simulink model "TLBO_2023"  (R2023b)
settings: Solver=ode45  StartTime=0.0  StopTime=6  MaxStep=1e-4  RelTol=1e-3  EnableMultiTasking=on
PreLoadFcn:
  | Ts_Power=1e-6;
  | Ts_Control=100e-6;
InitFcn:
  | Ts_Power=1e-6;
  | Ts_Control=100e-6;
  | Rtrans=0.142;
  | Xtrans=0.12e-6;
undefined symbols (not defined in the file): DiscIntNeverNeededParam, Ion, Lithium, sigbuilder_block
libraries: dspfdesign x80, spsSeriesRLCBranchLib x52, spsCurrentMeasurementLib x20, spsMeanLib x20, spsIdealSwitchLib x16, spsVoltageMeasurementLib x16, slpidlib x15, spsMosfetLib x14, dspindex x12, spsPWMGeneratorDCDCLib x10, spsGroundLib x10, spsBatteryLib x4
(part 1 of 4)
settings Model: Creator=Philip  LastModifiedBy=LEGION
settings SolverCC: AlgebraicLoopSolver=TrustRegion
settings DataIOCC: ReturnWorkspaceOutputs=off
settings OptimizationCC: LifeSpan=inf
settings DebuggingCC: UnconnectedInputMsg=warning  UnconnectedOutputMsg=warning  UnconnectedLineMsg=warning  SFUnexpectedBacktrackingDiag=warning  SFNoUnconditionalDefaultTransitionDiag=warning  SFExecutionAtInitializationDiag=none  UnderSpecifiedDimensionMsg=warning  ArithmeticOperatorsInVariantConditions=warning
settings ModelReferenceCC: EnableRefExpFcnMdlSchedulingChecks=on
settings SFSimCC: SimUseLocalCustomCode=off  CustomCodeUndefinedFunction=UseInterfaceOnly
settings RTWCC: RTWUseLocalCustomCode=off  DLArmComputeVersion=19.05
settings CodeAppCC: StateflowObjectComments=on
settings GRTTargetCC: TargetLangStandard=C89/C90 (ANSI)
settings ConfigComp: CovMetricSettings=dw  CovSaveCumulativeToWorkspaceVar=on  CovSaveSingleToWorkspaceVar=on  CovExternalEMLEnable=off
settings SimscapeCC: SimscapeNormalizeSystem=off

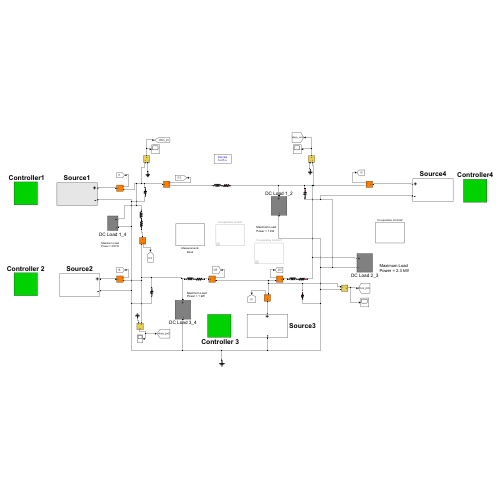
[thumbnail: Simulink's stored preview of the top-level diagram]
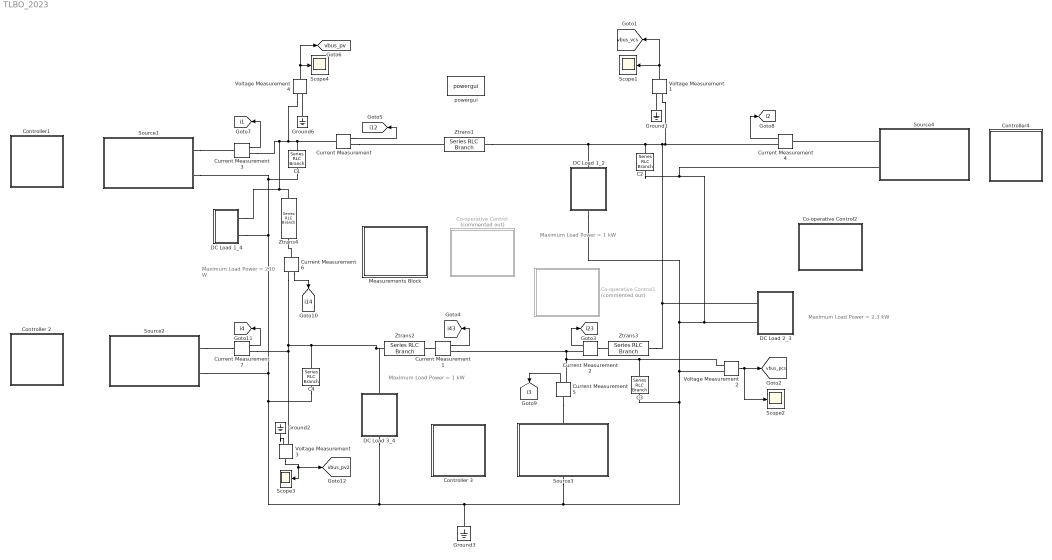
== system TLBO_2023 ==
  note: Maximum Load Power = 1 kW
  note: Maximum Load Power = 230 W
  note: Maximum Load Power = 2.3 kW
  note: Maximum Load Power = 1 kW
  " Controller 3" : Subsystem
  " Controller1" : Subsystem
  C{1..4} (4 alike) : spsSeriesRLCBranchLib/Series RLC Branch  LConnTagsString=__new0  RConnTagsString=__new0  BranchType=C  Resistance=1.0  Inductance=1.0  SetiL0=off  InitialCurrent=0  Capacitance=220e-6  Setx0=off  InitialVoltage=0  Measurements=Branch voltage
  Co-operative Control : Subsystem  Commented=on
  Co-operative Control1 : Subsystem  Commented=on
  Co-operative Control2 : Subsystem
  Controller 2 : Subsystem
  Controller4 : Subsystem
  Current Measurement{,1..7} (8 alike) : spsCurrentMeasurementLib/Current Measurement  PhasorSimulation=off  OutputType=Complex  PSBequivalent=0
  DC Load 1_2 : Subsystem
      settings: PortSchema="{\"entries\":[{\"content\":{\"sides\":[{\"content\":{\"connectorIds\":[]},\"type\":\"ConnectorPlacement.EquallySpacedRectSide\",\"uuid\":\"cddf6359-65bd-4051-86a6-0e07a89083cb\"},{\"content\":{\"connectorIds\":[],\"side\":\"RIGHT\"},\"type\":\"ConnectorPlacement.EquallySpacedRectSide\",\"uuid\":\"60c20b22-281d-4f49-a5be-0230fdaab524\"},{\"content\":{\"connectorIds\":[\"LConn1\"],\"side\":\"TOP\"},\"type\":\"ConnectorPlacement.EquallySpacedRectSide\",\"uuid\":\"1fa402d6-fa22-4172-ba4c-d6acb4a43f4e\"},{\"content\":{\"connectorIds\":[\"RConn1\"],\"side\":\"BOTTOM\"},\"type\":\"ConnectorPlacement.EquallySpacedRectSide\",\"uuid\":\"96e406b9-0d6c-4b79-8101-f8a8e2f9c4fc\"}]},\"type\":\"ConnectorPlacement.EquallySpacedConnector\",\"uuid\":\"d88be4f8-9f42-4009-a911-5cffa4248009\"}],\"packageUris\":[\"http://schema.mathworks.com/mf0/Connector/R2020b\"],\"version\":\"1.0\"}"
  DC Load 1_4 : Subsystem
  DC Load 2_3 : Subsystem
  DC Load 3_4 : Subsystem
      settings: PortSchema="{\"entries\":[{\"content\":{\"sides\":[{\"content\":{\"connectorIds\":[]},\"type\":\"ConnectorPlacement.EquallySpacedRectSide\",\"uuid\":\"cddf6359-65bd-4051-86a6-0e07a89083cb\"},{\"content\":{\"connectorIds\":[],\"side\":\"RIGHT\"},\"type\":\"ConnectorPlacement.EquallySpacedRectSide\",\"uuid\":\"60c20b22-281d-4f49-a5be-0230fdaab524\"},{\"content\":{\"connectorIds\":[\"LConn1\"],\"side\":\"TOP\"},\"type\":\"ConnectorPlacement.EquallySpacedRectSide\",\"uuid\":\"1fa402d6-fa22-4172-ba4c-d6acb4a43f4e\"},{\"content\":{\"connectorIds\":[\"RConn1\"],\"side\":\"BOTTOM\"},\"type\":\"ConnectorPlacement.EquallySpacedRectSide\",\"uuid\":\"96e406b9-0d6c-4b79-8101-f8a8e2f9c4fc\"}]},\"type\":\"ConnectorPlacement.EquallySpacedConnector\",\"uuid\":\"d88be4f8-9f42-4009-a911-5cffa4248009\"}],\"packageUris\":[\"http://schema.mathworks.com/mf0/Connector/R2020b\"],\"version\":\"1.0\"}"
  Ground{1..3,6} (4 alike) : spsGroundLib/Ground  LConnTagsString=a
  Measurements Block : Subsystem
  Scope{1..4} (4 alike) : Scope
  Source1 : Subsystem
  Source2 : Subsystem
  Source3 : Subsystem
  Source4 : Subsystem
  Voltage Measurement{1..4} (4 alike) : spsVoltageMeasurementLib/Voltage Measurement  PhasorSimulation=off  OutputType=Complex  PSBequivalent=0
  Ztrans{1..4} (4 alike) : spsSeriesRLCBranchLib/Series RLC Branch  LConnTagsString=__new0  RConnTagsString=__new0  BranchType=RL  Resistance=Rtrans  Inductance=Xtrans  SetiL0=off  InitialCurrent=0  Capacitance=220e-6  Setx0=off  InitialVoltage=0  Measurements=None
  powergui : spspowerguiLib/powergui  Priority=1  SimulationMode=Discrete  SampleTime=1e-5  frequency=60  Iterations=50  frequencyindice=0  Pbase=100e6  ErrMax=1e-4  UnitsV=kV  UnitsW=MW  buscounter=0  FunctionMessages=off  echomessages=off  EnableUseOfTLC=off  CurrentSourceSwitches=off  DisableSnubberDevices=off  DisableRonSwitches=off  DisableVfSwitches=off  DisplayEquations=off  AutomaticDiscreteSolvers=off  SolverType=Tustin/Backward Euler (TBE)  Interpol=off  ExternalGateDelay=off  methode=off  Ts=100  x0status=blocks  SPID=on  SwTol=0  HookPort=off  NonlinearTolerance=1e-4  nMaxIteration=100  ContinueOnMaxIteration=off  RestoreLinks=warning  ResistiveCurrentMeasurement=off  Frange=[0:2:500]  Ylog=off  Xlog=on  ShowGrid=off  save=off  variable=ZData  structure=0  ZoomFFT=off  StartTime=0.0  cycles=1  DisplayStyle=1  fundamental=60  FreqAxis=off  MaxFrequency=1000  frequencyindicesteady=1  RmsSteady=1  display=off
  tag scope: i12=global, i14=global, i1=global, i23=global, i2=global, i3=global, i43=global, i4=global, vbus_pcs=global, vbus_pv2=global, vbus_pv=global, vbus_vcs=global
  wires:
  Voltage Measurement4/1 -> [vbus_pv], Scope4/1
  Voltage Measurement1/1 -> [vbus_vcs], Scope1/1
  Current Measurement2/1 -> [i23]
  Current Measurement1/1 -> [i43]
  Current Measurement/1 -> [i12]
  Voltage Measurement2/1 -> Scope2/1, [vbus_pcs]
  Current Measurement3/1 -> [i1]
  Current Measurement5/1 -> [i3]
  Current Measurement6/1 -> [i14]
  Current Measurement7/1 -> [i4]
  Voltage Measurement3/1 -> Scope3/1, [vbus_pv2]
  Current Measurement4/1 -> [i2]
  connections:
  Source4/RConn2 -- C2/RConn1 -- Source3/LConn1 -- Ground3/LConn1 -- C4/RConn1 -- C1/RConn1 -- Source1/RConn2 -- DC Load 1_4/LConn2 -- Source2/RConn2 -- DC Load 3_4/RConn1 -- C3/RConn1 -- Voltage Measurement2/LConn2 -- DC Load 1_2/RConn1 -- DC Load 2_3/LConn2
  DC Load 2_3/LConn1 -- Current Measurement4/RConn1 -- Voltage Measurement1/LConn1 -- Ztrans1/LConn1 -- DC Load 1_2/LConn1 -- C2/LConn1 -- Ztrans3/LConn1
  C3/LConn1 -- Voltage Measurement2/LConn1 -- Current Measurement1/RConn1 -- Current Measurement2/RConn1 -- Current Measurement5/RConn1
  Ground6/LConn1 -- Voltage Measurement4/LConn2
  Ground1/LConn1 -- Voltage Measurement1/LConn2
  Current Measurement/RConn1 -- Ztrans1/RConn1
  Current Measurement1/LConn1 -- Ztrans2/LConn1
  Ztrans3/RConn1 -- Current Measurement2/LConn1
  Source1/RConn1 -- Current Measurement3/LConn1
  Source4/RConn1 -- Current Measurement4/LConn1
  Current Measurement5/LConn1 -- Source3/RConn1
  Current Measurement3/RConn1 -- Voltage Measurement4/LConn1 -- Current Measurement/LConn1 -- C1/LConn1 -- Ztrans4/RConn1 -- DC Load 1_4/LConn1
  Current Measurement7/RConn1 -- DC Load 3_4/LConn1 -- Ztrans2/RConn1 -- C4/LConn1 -- Current Measurement6/RConn1 -- Voltage Measurement3/LConn1
  Source2/RConn1 -- Current Measurement7/LConn1
  Ground2/LConn1 -- Voltage Measurement3/LConn2
  Current Measurement6/LConn1 -- Ztrans4/LConn1

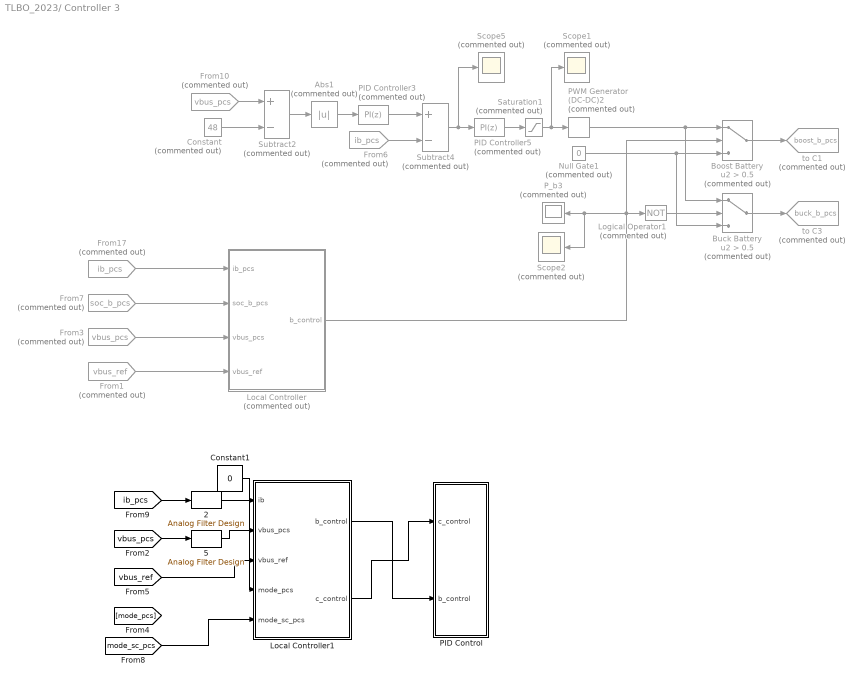
== system TLBO_2023/ Controller 3 ==
  2 : dspfdesign/Analog Filter Design  method=Butterworth  filttype=Lowpass  N=8  Wlo=pi*50  Whi=80  Rp=2  Rs=40
  5 : dspfdesign/Analog Filter Design  method=Butterworth  filttype=Lowpass  N=8  Wlo=pi*50  Whi=80  Rp=2  Rs=40
  Abs1 : Abs  Commented=on  SaturateOnIntegerOverflow=off
  Boost Battery : Switch  Commented=on  Criteria=u2 > Threshold  Threshold=0.5  SaturateOnIntegerOverflow=off  InputSameDT=off
  Buck Battery : Switch  Commented=on  Criteria=u2 > Threshold  Threshold=0.5  SaturateOnIntegerOverflow=off  InputSameDT=off
  Constant : Constant  Commented=on  Value=48
  Constant1 : Constant  Value=0
  From1 : From  Commented=on  GotoTag=vbus_ref  TagVisibility=global
  From10 : From  Commented=on  GotoTag=vbus_pcs  TagVisibility=global
  From17 : From  Commented=on  GotoTag=ib_pcs  TagVisibility=global
  From3 : From  Commented=on  GotoTag=vbus_pcs  TagVisibility=global
  From6 : From  Commented=on  GotoTag=ib_pcs  TagVisibility=global
  From7 : From  Commented=on  GotoTag=soc_b_pcs  TagVisibility=global
  Local Controller : MATLAB Function  Commented=on  TreatAsAtomicUnit=on
  Local Controller1 : MATLAB Function  TreatAsAtomicUnit=on
  Logical Operator1 : Logic  Commented=on  Operator=NOT  AllPortsSameDT=off  OutDataTypeStr=boolean
  Null Gate1 : Constant  Commented=on  Value=0
  PID Control : Subsystem
  PID Controller3 : slpidlib/PID Controller  Commented=on  Controller=PI  Form=Parallel  TimeDomain=Discrete-time  UseExternalTs=off  SampleTime=-1  IntegratorMethod=Forward Euler  FilterMethod=Forward Euler  ControllerParametersSource=internal  P=0  I=4  UseKiTs=off  D=0  N=100  UseFilter=on  TunerSelectOption=Transfer Function Based (PID Tuner App)  InitialConditionSource=internal  InitialConditionForIntegrator=0  InitialConditionForFilter=0  DifferentiatorICPrevScaledInput=0  ExternalReset=none  TrackingMode=off  Kt=1  LimitOutput=off  SatLimitsSource=internal  UpperSaturationLimit=inf  LowerSaturationLimit=-inf  LinearizeAsGain=on  AntiWindupMode=none  Kb=1  LimitIntegrator=off  UpperIntegratorSaturationLimit=inf  LowerIntegratorSaturationLimit=-inf  POutMin=[]  POutMax=[]  IOutMin=[]  IOutMax=[]  DOutMin=[]  DOutMax=[]  NOutMin=[]  NOutMax=[]  SumOutMin=[]  SumOutMax=[]  SaturationOutMin=[]  SaturationOutMax=[]  PParamMin=[]  PParamMax=[]  IParamMin=[]  IParamMax=[]  DParamMin=[]  DParamMax=[]  NParamMin=[]  NParamMax=[]  KbParamMin=[]  KbParamMax=[]  KtParamMin=[]  KtParamMax=[]  KbOutMin=[]  KbOutMax=[]  KtOutMin=[]  KtOutMax=[]  IntegratorOutMin=[]  IntegratorOutMax=[]  FilterOutMin=[]  FilterOutMax=[]  SumI1OutMin=[]  SumI1OutMax=[]  SumI2OutMin=[]  SumI2OutMax=[]  SumI3OutMin=[]  SumI3OutMax=[]  SumI4OutMin=[]  SumI4OutMax=[]  SumDOutMin=[]  SumDOutMax=[]  DifferentiatorOutMin=[]  DifferentiatorOutMax=[]  FilterDiffOutCoefMin=[]  FilterDiffOutCoefMax=[]  ReciprocalOutMin=[]  ReciprocalOutMax=[]  SumDenOutMin=[]  SumDenOutMax=[]  SumNumOutMin=[]  SumNumOutMax=[]  DivideOutMin=[]  DivideOutMax=[]  UdiffTsProdOutMin=[]  UdiffTsProdOutMax=[]  NTsProdOutMin=[]  NTsProdOutMax=[]  UintegralTsProdOutMin=[]  UintegralTsProdOutMax=[]  UngainTsProdOutMin=[]  UngainTsProdOutMax=[]  ClampingZeroOutDataTypeStr=Inherit: Inherit via back propagation  ClampingZeroOutMin=[]  ClampingZeroOutMax=[]  FilterDenConstantOutDataTypeStr=Inherit: Inherit via back propagation  FilterDenConstantOutMin=[]  FilterDenConstantOutMax=[]  PCopyOutDataTypeStr=Inherit: Inherit via back propagation  PCopyOutMin=[]  PCopyOutMax=[]  NCopyOutDataTypeStr=Inherit: Inherit via back propagation  NCopyOutMin=[]  NCopyOutMax=[]  IntegratorContinuousStateAttributes=''  IntegratorStateMustResolveToSignalObject=off  IntegratorRTWStateStorageClass=Auto  FilterContinuousStateAttributes=''  FilterStateMustResolveToSignalObject=off  FilterRTWStateStorageClass=Auto  ParallelPVariant=InternalParameters  IdealPVariant=Disabled  IVariant=InternalParameters  DVariant=Disabled  IntegratorVariant=Discrete  SatVariant=Disabled  AWVariant=Passthrough  PCopyVariant=Disabled  TRVariant=Disabled  FdbkBlocksVariant=Forward  IdealPFdbkVariant=Disabled  SatFdbkVariant=Disabled  DerivativeFilterVariant=Disabled  NVariant=Disabled  NCopyVariant=Disabled_SignalSpec  FilterICVariant=Disabled  IntegratorICVariant=InternalICs  ExternalResetVariant=Disabled  TRSumVariant=Passthrough  SumFdbkVariant=Disabled  SumVariant=Sum_PI  TsampFilterVariant=InternalTs  TsampNgainVariant=Passthrough  TsampIntegralVariant=Disabled_SignalSpec  ExternalSaturationOutDataTypeStr=Inherit: Same as second input
  PID Controller5 : slpidlib/PID Controller  Commented=on  Controller=PI  Form=Parallel  TimeDomain=Discrete-time  UseExternalTs=off  SampleTime=-1  IntegratorMethod=Forward Euler  FilterMethod=Forward Euler  ControllerParametersSource=internal  P=1  I=4  UseKiTs=off  D=1  N=100  UseFilter=on  TunerSelectOption=Transfer Function Based (PID Tuner App)  InitialConditionSource=internal  InitialConditionForIntegrator=0  InitialConditionForFilter=0  DifferentiatorICPrevScaledInput=0  ExternalReset=none  TrackingMode=off  Kt=1  LimitOutput=off  SatLimitsSource=internal  UpperSaturationLimit=inf  LowerSaturationLimit=-inf  LinearizeAsGain=on  AntiWindupMode=none  Kb=1  LimitIntegrator=off  UpperIntegratorSaturationLimit=inf  LowerIntegratorSaturationLimit=-inf  POutMin=[]  POutMax=[]  IOutMin=[]  IOutMax=[]  DOutMin=[]  DOutMax=[]  NOutMin=[]  NOutMax=[]  SumOutMin=[]  SumOutMax=[]  SaturationOutMin=[]  SaturationOutMax=[]  PParamMin=[]  PParamMax=[]  IParamMin=[]  IParamMax=[]  DParamMin=[]  DParamMax=[]  NParamMin=[]  NParamMax=[]  KbParamMin=[]  KbParamMax=[]  KtParamMin=[]  KtParamMax=[]  KbOutMin=[]  KbOutMax=[]  KtOutMin=[]  KtOutMax=[]  IntegratorOutMin=[]  IntegratorOutMax=[]  FilterOutMin=[]  FilterOutMax=[]  SumI1OutMin=[]  SumI1OutMax=[]  SumI2OutMin=[]  SumI2OutMax=[]  SumI3OutMin=[]  SumI3OutMax=[]  SumI4OutMin=[]  SumI4OutMax=[]  SumDOutMin=[]  SumDOutMax=[]  DifferentiatorOutMin=[]  DifferentiatorOutMax=[]  FilterDiffOutCoefMin=[]  FilterDiffOutCoefMax=[]  ReciprocalOutMin=[]  ReciprocalOutMax=[]  SumDenOutMin=[]  SumDenOutMax=[]  SumNumOutMin=[]  SumNumOutMax=[]  DivideOutMin=[]  DivideOutMax=[]  UdiffTsProdOutMin=[]  UdiffTsProdOutMax=[]  NTsProdOutMin=[]  NTsProdOutMax=[]  UintegralTsProdOutMin=[]  UintegralTsProdOutMax=[]  UngainTsProdOutMin=[]  UngainTsProdOutMax=[]  ClampingZeroOutDataTypeStr=Inherit: Inherit via back propagation  ClampingZeroOutMin=[]  ClampingZeroOutMax=[]  FilterDenConstantOutDataTypeStr=Inherit: Inherit via back propagation  FilterDenConstantOutMin=[]  FilterDenConstantOutMax=[]  PCopyOutDataTypeStr=Inherit: Inherit via back propagation  PCopyOutMin=[]  PCopyOutMax=[]  NCopyOutDataTypeStr=Inherit: Inherit via back propagation  NCopyOutMin=[]  NCopyOutMax=[]  IntegratorContinuousStateAttributes=''  IntegratorStateMustResolveToSignalObject=off  IntegratorRTWStateStorageClass=Auto  FilterContinuousStateAttributes=''  FilterStateMustResolveToSignalObject=off  FilterRTWStateStorageClass=Auto  ParallelPVariant=InternalParameters  IdealPVariant=Disabled  IVariant=InternalParameters  DVariant=Disabled  IntegratorVariant=Discrete  SatVariant=Disabled  AWVariant=Passthrough  PCopyVariant=Disabled  TRVariant=Disabled  FdbkBlocksVariant=Forward  IdealPFdbkVariant=Disabled  SatFdbkVariant=Disabled  DerivativeFilterVariant=Disabled  NVariant=Disabled  NCopyVariant=Disabled_SignalSpec  FilterICVariant=Disabled  IntegratorICVariant=InternalICs  ExternalResetVariant=Disabled  TRSumVariant=Passthrough  SumFdbkVariant=Disabled  SumVariant=Sum_PI  TsampFilterVariant=InternalTs  TsampNgainVariant=Passthrough  TsampIntegralVariant=Disabled_SignalSpec  ExternalSaturationOutDataTypeStr=Inherit: Same as second input
  PWM Generator (DC-DC)2 : spsPWMGeneratorDCDCLib/PWM Generator (DC-DC)  Commented=on  Fsw=10e3  Ts=0
  P_b3 : Display  Commented=on
      settings: Format=binary (Stored Integer)  Decimation=1000
  Saturation1 : Saturate  Commented=on  UpperLimit=0.8  LowerLimit=0  ZeroCross=off
  Scope1 : Scope  Commented=on
  Scope2 : Scope  Commented=on
  Scope5 : Scope  Commented=on
  Subtract2 : Sum  Commented=on  Inputs=+-
  Subtract4 : Sum  Commented=on  Inputs=+-
  to C1 : Goto  Commented=on  GotoTag=boost_b_pcs  TagVisibility=global
  to C3 : Goto  Commented=on  GotoTag=buck_b_pcs  TagVisibility=global
  wires:
  Constant/1 -> Subtract2/2
  From1/1 -> Local Controller/4(vbus_ref)
  From6/1 -> Subtract4/2
  PID Controller3/1 -> Subtract4/1
  Subtract4/1 -> PID Controller5/1, Scope5/1
  Saturation1/1 -> PWM Generator (DC-DC)2/1, Scope1/1
  PID Controller5/1 -> Saturation1/1
  PWM Generator (DC-DC)2/1 -> Boost Battery/1, Buck Battery/1
  Abs1/1 -> PID Controller3/1
  From10/1 -> Subtract2/1
  Local Controller/1(b_control) -> Boost Battery/2, Logical Operator1/1, P_b3/1, Scope2/1
  Logical Operator1/1 -> Buck Battery/2
  Subtract2/1 -> Abs1/1
  From7/1 -> Local Controller/2(soc_b_pcs)
  From3/1 -> Local Controller/3(vbus_pcs)
  From17/1 -> Local Controller/1(ib_pcs)
  Null Gate1/1 -> Buck Battery/3, Boost Battery/3
  Boost Battery/1 -> to C1/1
  Buck Battery/1 -> to C3/1
  [vbus_pcs] -> 5/1
  [ib_pcs] -> 2/1
  2/1 -> Local Controller1/1(ib)
  5/1 -> Local Controller1/2(vbus_pcs)
  [vbus_ref] -> Local Controller1/3(vbus_ref)
  Local Controller1/1(b_control) -> PID Control/2(b_control)
  Local Controller1/2(c_control) -> PID Control/1(c_control)
  [mode_sc_pcs] -> Local Controller1/5(mode_sc_pcs)
  Constant1/1 -> Local Controller1/4(mode_pcs)

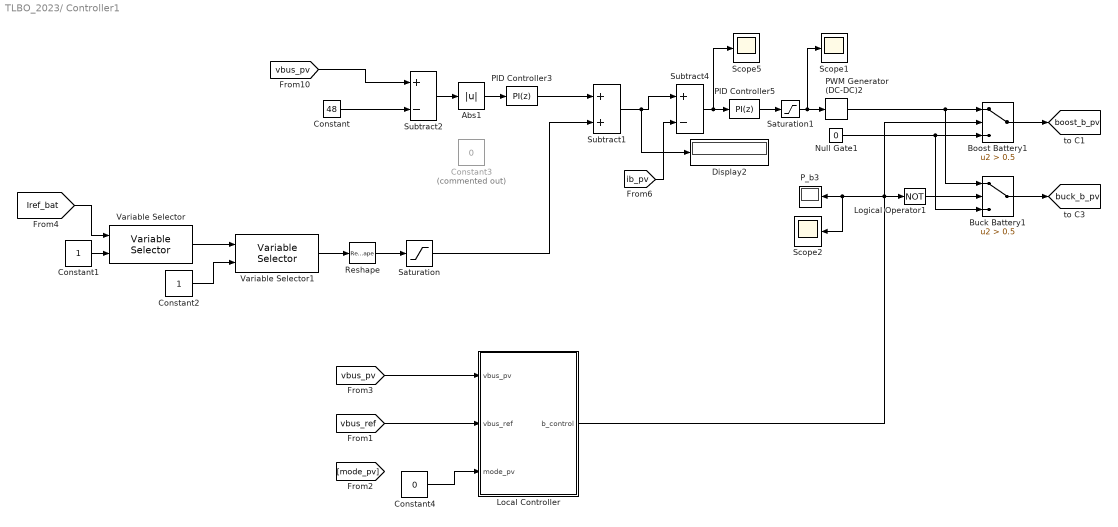
== system TLBO_2023/ Controller1 ==
  Abs1 : Abs  SaturateOnIntegerOverflow=off
  Boost Battery1 : Switch  Criteria=u2 > Threshold  Threshold=0.5  SaturateOnIntegerOverflow=off  InputSameDT=off
  Buck Battery1 : Switch  Criteria=u2 > Threshold  Threshold=0.5  SaturateOnIntegerOverflow=off  InputSameDT=off
  Constant : Constant  Value=48
  Constant1 : Constant
  Constant2 : Constant
  Constant3 : Constant  Commented=on  Value=0
  Constant4 : Constant  Value=0
  Display2 : Display
  Local Controller : MATLAB Function  TreatAsAtomicUnit=on
  Logical Operator1 : Logic  Operator=NOT  AllPortsSameDT=off  OutDataTypeStr=boolean
  Null Gate1 : Constant  Value=0
  PID Controller3 : slpidlib/PID Controller  Controller=PI  Form=Parallel  TimeDomain=Discrete-time  UseExternalTs=off  SampleTime=-1  IntegratorMethod=Forward Euler  FilterMethod=Forward Euler  ControllerParametersSource=internal  P=0  I=4  UseKiTs=off  D=0  N=100  UseFilter=on  TunerSelectOption=Transfer Function Based (PID Tuner App)  InitialConditionSource=internal  InitialConditionForIntegrator=0  InitialConditionForFilter=0  DifferentiatorICPrevScaledInput=0  ExternalReset=none  TrackingMode=off  Kt=1  LimitOutput=off  SatLimitsSource=internal  UpperSaturationLimit=inf  LowerSaturationLimit=-inf  LinearizeAsGain=on  AntiWindupMode=none  Kb=1  LimitIntegrator=off  UpperIntegratorSaturationLimit=inf  LowerIntegratorSaturationLimit=-inf  POutMin=[]  POutMax=[]  IOutMin=[]  IOutMax=[]  DOutMin=[]  DOutMax=[]  NOutMin=[]  NOutMax=[]  SumOutMin=[]  SumOutMax=[]  SaturationOutMin=[]  SaturationOutMax=[]  PParamMin=[]  PParamMax=[]  IParamMin=[]  IParamMax=[]  DParamMin=[]  DParamMax=[]  NParamMin=[]  NParamMax=[]  KbParamMin=[]  KbParamMax=[]  KtParamMin=[]  KtParamMax=[]  KbOutMin=[]  KbOutMax=[]  KtOutMin=[]  KtOutMax=[]  IntegratorOutMin=[]  IntegratorOutMax=[]  FilterOutMin=[]  FilterOutMax=[]  SumI1OutMin=[]  SumI1OutMax=[]  SumI2OutMin=[]  SumI2OutMax=[]  SumI3OutMin=[]  SumI3OutMax=[]  SumI4OutMin=[]  SumI4OutMax=[]  SumDOutMin=[]  SumDOutMax=[]  DifferentiatorOutMin=[]  DifferentiatorOutMax=[]  FilterDiffOutCoefMin=[]  FilterDiffOutCoefMax=[]  ReciprocalOutMin=[]  ReciprocalOutMax=[]  SumDenOutMin=[]  SumDenOutMax=[]  SumNumOutMin=[]  SumNumOutMax=[]  DivideOutMin=[]  DivideOutMax=[]  UdiffTsProdOutMin=[]  UdiffTsProdOutMax=[]  NTsProdOutMin=[]  NTsProdOutMax=[]  UintegralTsProdOutMin=[]  UintegralTsProdOutMax=[]  UngainTsProdOutMin=[]  UngainTsProdOutMax=[]  ClampingZeroOutDataTypeStr=Inherit: Inherit via back propagation  ClampingZeroOutMin=[]  ClampingZeroOutMax=[]  FilterDenConstantOutDataTypeStr=Inherit: Inherit via back propagation  FilterDenConstantOutMin=[]  FilterDenConstantOutMax=[]  PCopyOutDataTypeStr=Inherit: Inherit via back propagation  PCopyOutMin=[]  PCopyOutMax=[]  NCopyOutDataTypeStr=Inherit: Inherit via back propagation  NCopyOutMin=[]  NCopyOutMax=[]  IntegratorContinuousStateAttributes=''  IntegratorStateMustResolveToSignalObject=off  IntegratorRTWStateStorageClass=Auto  FilterContinuousStateAttributes=''  FilterStateMustResolveToSignalObject=off  FilterRTWStateStorageClass=Auto  ParallelPVariant=InternalParameters  IdealPVariant=Disabled  IVariant=InternalParameters  DVariant=Disabled  IntegratorVariant=Discrete  SatVariant=Disabled  AWVariant=Passthrough  PCopyVariant=Disabled  TRVariant=Disabled  FdbkBlocksVariant=Forward  IdealPFdbkVariant=Disabled  SatFdbkVariant=Disabled  DerivativeFilterVariant=Disabled  NVariant=Disabled  NCopyVariant=Disabled_SignalSpec  FilterICVariant=Disabled  IntegratorICVariant=InternalICs  ExternalResetVariant=Disabled  TRSumVariant=Passthrough  SumFdbkVariant=Disabled  SumVariant=Sum_PI  TsampFilterVariant=InternalTs  TsampNgainVariant=Passthrough  TsampIntegralVariant=Disabled_SignalSpec  ExternalSaturationOutDataTypeStr=Inherit: Same as second input
  PID Controller5 : slpidlib/PID Controller  Controller=PI  Form=Parallel  TimeDomain=Discrete-time  UseExternalTs=off  SampleTime=-1  IntegratorMethod=Forward Euler  FilterMethod=Forward Euler  ControllerParametersSource=internal  P=10  I=4  UseKiTs=off  D=10  N=100  UseFilter=on  TunerSelectOption=Transfer Function Based (PID Tuner App)  InitialConditionSource=internal  InitialConditionForIntegrator=0  InitialConditionForFilter=0  DifferentiatorICPrevScaledInput=0  ExternalReset=none  TrackingMode=off  Kt=1  LimitOutput=off  SatLimitsSource=internal  UpperSaturationLimit=inf  LowerSaturationLimit=-inf  LinearizeAsGain=on  AntiWindupMode=none  Kb=1  LimitIntegrator=off  UpperIntegratorSaturationLimit=inf  LowerIntegratorSaturationLimit=-inf  POutMin=[]  POutMax=[]  IOutMin=[]  IOutMax=[]  DOutMin=[]  DOutMax=[]  NOutMin=[]  NOutMax=[]  SumOutMin=[]  SumOutMax=[]  SaturationOutMin=[]  SaturationOutMax=[]  PParamMin=[]  PParamMax=[]  IParamMin=[]  IParamMax=[]  DParamMin=[]  DParamMax=[]  NParamMin=[]  NParamMax=[]  KbParamMin=[]  KbParamMax=[]  KtParamMin=[]  KtParamMax=[]  KbOutMin=[]  KbOutMax=[]  KtOutMin=[]  KtOutMax=[]  IntegratorOutMin=[]  IntegratorOutMax=[]  FilterOutMin=[]  FilterOutMax=[]  SumI1OutMin=[]  SumI1OutMax=[]  SumI2OutMin=[]  SumI2OutMax=[]  SumI3OutMin=[]  SumI3OutMax=[]  SumI4OutMin=[]  SumI4OutMax=[]  SumDOutMin=[]  SumDOutMax=[]  DifferentiatorOutMin=[]  DifferentiatorOutMax=[]  FilterDiffOutCoefMin=[]  FilterDiffOutCoefMax=[]  ReciprocalOutMin=[]  ReciprocalOutMax=[]  SumDenOutMin=[]  SumDenOutMax=[]  SumNumOutMin=[]  SumNumOutMax=[]  DivideOutMin=[]  DivideOutMax=[]  UdiffTsProdOutMin=[]  UdiffTsProdOutMax=[]  NTsProdOutMin=[]  NTsProdOutMax=[]  UintegralTsProdOutMin=[]  UintegralTsProdOutMax=[]  UngainTsProdOutMin=[]  UngainTsProdOutMax=[]  ClampingZeroOutDataTypeStr=Inherit: Inherit via back propagation  ClampingZeroOutMin=[]  ClampingZeroOutMax=[]  FilterDenConstantOutDataTypeStr=Inherit: Inherit via back propagation  FilterDenConstantOutMin=[]  FilterDenConstantOutMax=[]  PCopyOutDataTypeStr=Inherit: Inherit via back propagation  PCopyOutMin=[]  PCopyOutMax=[]  NCopyOutDataTypeStr=Inherit: Inherit via back propagation  NCopyOutMin=[]  NCopyOutMax=[]  IntegratorContinuousStateAttributes=''  IntegratorStateMustResolveToSignalObject=off  IntegratorRTWStateStorageClass=Auto  FilterContinuousStateAttributes=''  FilterStateMustResolveToSignalObject=off  FilterRTWStateStorageClass=Auto  ParallelPVariant=InternalParameters  IdealPVariant=Disabled  IVariant=InternalParameters  DVariant=Disabled  IntegratorVariant=Discrete  SatVariant=Disabled  AWVariant=Passthrough  PCopyVariant=Disabled  TRVariant=Disabled  FdbkBlocksVariant=Forward  IdealPFdbkVariant=Disabled  SatFdbkVariant=Disabled  DerivativeFilterVariant=Disabled  NVariant=Disabled  NCopyVariant=Disabled_SignalSpec  FilterICVariant=Disabled  IntegratorICVariant=InternalICs  ExternalResetVariant=Disabled  TRSumVariant=Passthrough  SumFdbkVariant=Disabled  SumVariant=Sum_PI  TsampFilterVariant=InternalTs  TsampNgainVariant=Passthrough  TsampIntegralVariant=Disabled_SignalSpec  ExternalSaturationOutDataTypeStr=Inherit: Same as second input
  PWM Generator (DC-DC)2 : spsPWMGeneratorDCDCLib/PWM Generator (DC-DC)  Fsw=10e3  Ts=0
  P_b3 : Display
      settings: Format=binary (Stored Integer)  Decimation=1000
  Reshape : Reshape
  Saturation : Saturate
  Saturation1 : Saturate  UpperLimit=0.8  LowerLimit=0  ZeroCross=off
  Scope1 : Scope
  Scope2 : Scope
  Scope5 : Scope
  Subtract1 : Sum
  Subtract2 : Sum  Inputs=+-
  Subtract4 : Sum  Inputs=+-
  Variable Selector : dspindex/Variable Selector  NumInputs=1  rowsOrCols=Rows  IdxMode=Variable  Elements=[1 3]  ZerOneIdxMode=One-based  errmode=Clip Index  FillMode=on  FillValues=0
  Variable Selector1 : dspindex/Variable Selector  NumInputs=1  rowsOrCols=Columns  IdxMode=Variable  Elements=[1 3]  ZerOneIdxMode=One-based  errmode=Clip Index  FillMode=on  FillValues=0
  tag scope: boost_b_pv=global, buck_b_pv=global
  wires:
  Buck Battery1/1 -> [buck_b_pv]
  Boost Battery1/1 -> [boost_b_pv]
  Null Gate1/1 -> Boost Battery1/3, Buck Battery1/3
  [vbus_pv] -> Local Controller/1(vbus_pv)
  Subtract2/1 -> Abs1/1
  Logical Operator1/1 -> Buck Battery1/2
  Local Controller/1(b_control) -> Scope2/1, P_b3/1, Logical Operator1/1, Boost Battery1/2
  Abs1/1 -> PID Controller3/1
  PWM Generator (DC-DC)2/1 -> Buck Battery1/1, Boost Battery1/1
  PID Controller5/1 -> Saturation1/1
  Saturation1/1 -> Scope1/1, PWM Generator (DC-DC)2/1
  Subtract4/1 -> Scope5/1, PID Controller5/1
  [vbus_ref] -> Local Controller/2(vbus_ref)
  [ib_pv] -> Subtract4/2
  [vbus_pv] -> Subtract2/1
  [Iref_bat] -> Variable Selector/1
  Constant1/1 -> Variable Selector/2
  Variable Selector/1 -> Variable Selector1/1
  Constant2/1 -> Variable Selector1/2
  Constant/1 -> Subtract2/2
  Variable Selector1/1 -> Reshape/1
  PID Controller3/1 -> Subtract1/1
  Subtract1/1 -> Display2/1, Subtract4/1
  Reshape/1 -> Saturation/1
  Saturation/1 -> Subtract1/2
  Constant4/1 -> Local Controller/3(mode_pv)

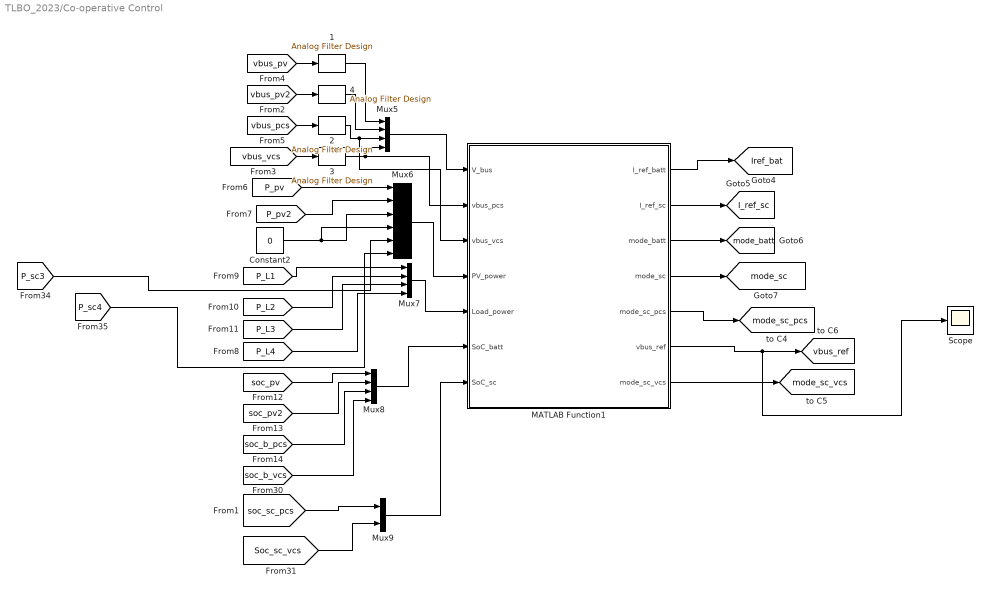
== system TLBO_2023/Co-operative Control ==
  {1..4} (4 alike) : dspfdesign/Analog Filter Design  method=Butterworth  filttype=Lowpass  N=8  Wlo=pi*50  Whi=80  Rp=2  Rs=40
  Constant2 : Constant  Value=0
  MATLAB Function1 : MATLAB Function  TreatAsAtomicUnit=on
  Mux5 : Mux
  Mux6 : Mux  Inputs=6
  Mux7 : Mux
  Mux8 : Mux
  Mux9 : Mux  Inputs=2
  Scope : Scope
  tag scope: I_ref_sc=global, Iref_bat=global, mode_batt=global, mode_sc=global, mode_sc_pcs=global, mode_sc_vcs=global, vbus_ref=global
  wires:
  Mux5/1 -> MATLAB Function1/1(V_bus)
  [P_L1] -> Mux7/1
  [Soc_sc_vcs] -> Mux9/2
  Constant2/1 -> Mux6/3, Mux6/4
  [P_pv2] -> Mux6/2
  Mux8/1 -> MATLAB Function1/6(SoC_batt)
  [soc_b_vcs] -> Mux8/4
  [vbus_pv2] -> 4/1
  [P_pv] -> Mux6/1
  [soc_pv2] -> Mux8/2
  [vbus_vcs] -> 3/1
  2/1 -> MATLAB Function1/3(vbus_vcs), Mux5/3
  [vbus_pcs] -> 2/1
  [soc_sc_pcs] -> Mux9/1
  [P_L3] -> Mux7/3
  3/1 -> MATLAB Function1/2(vbus_pcs), Mux5/4
  [vbus_pv] -> 1/1
  Mux9/1 -> MATLAB Function1/7(SoC_sc)
  [P_L2] -> Mux7/2
  [soc_b_pcs] -> Mux8/3
  1/1 -> Mux5/1
  [soc_pv] -> Mux8/1
  Mux6/1 -> MATLAB Function1/4(PV_power)
  Mux7/1 -> MATLAB Function1/5(Load_power)
  [P_L4] -> Mux7/4
  4/1 -> Mux5/2
  MATLAB Function1/1(I_ref_batt) -> [Iref_bat]
  [P_sc4] -> Mux6/6
  [P_sc3] -> Mux6/5
  MATLAB Function1/2(I_ref_sc) -> [I_ref_sc]
  MATLAB Function1/3(mode_batt) -> [mode_batt]
  MATLAB Function1/4(mode_sc) -> [mode_sc]
  MATLAB Function1/5(mode_sc_pcs) -> [mode_sc_pcs]
  MATLAB Function1/7(mode_sc_vcs) -> [mode_sc_vcs]
  MATLAB Function1/6(vbus_ref) -> Scope/1, [vbus_ref]

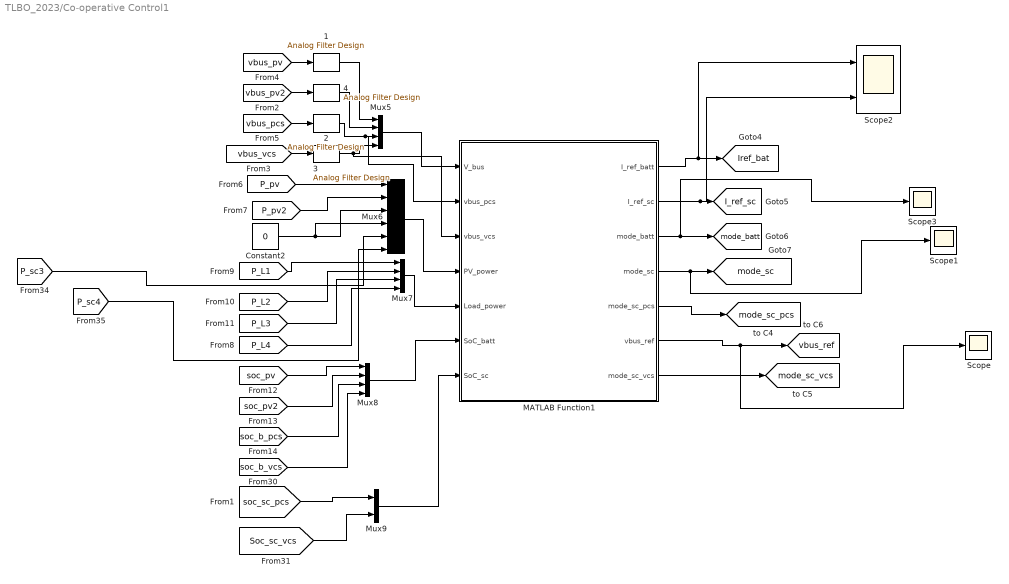
== system TLBO_2023/Co-operative Control1 ==
  {1..4} (4 alike) : dspfdesign/Analog Filter Design  method=Butterworth  filttype=Lowpass  N=8  Wlo=pi*50  Whi=80  Rp=2  Rs=40
  Constant2 : Constant  Value=0
  MATLAB Function1 : MATLAB Function  TreatAsAtomicUnit=on
  Mux5 : Mux
  Mux6 : Mux  Inputs=6
  Mux7 : Mux
  Mux8 : Mux
  Mux9 : Mux  Inputs=2
  Scope : Scope
  Scope1 : Scope
  Scope2 : Scope  NumInputPorts=2
  Scope3 : Scope
  tag scope: I_ref_sc=global, Iref_bat=global, mode_batt=global, mode_sc=global, mode_sc_pcs=global, mode_sc_vcs=global, vbus_ref=global
  wires:
  MATLAB Function1/6(vbus_ref) -> Scope/1, [vbus_ref]
  MATLAB Function1/7(mode_sc_vcs) -> [mode_sc_vcs]
  MATLAB Function1/5(mode_sc_pcs) -> [mode_sc_pcs]
  MATLAB Function1/4(mode_sc) -> Scope1/1, [mode_sc]
  MATLAB Function1/3(mode_batt) -> Scope3/1, [mode_batt]
  MATLAB Function1/2(I_ref_sc) -> Scope2/2, [I_ref_sc]
  [P_sc3] -> Mux6/5
  [P_sc4] -> Mux6/6
  MATLAB Function1/1(I_ref_batt) -> Scope2/1, [Iref_bat]
  4/1 -> Mux5/2
  [P_L4] -> Mux7/4
  [soc_pv] -> Mux8/1
  1/1 -> Mux5/1
  [soc_b_pcs] -> Mux8/3
  [P_L2] -> Mux7/2
  [vbus_pv] -> 1/1
  3/1 -> MATLAB Function1/3(vbus_vcs), Mux5/4
  [P_L3] -> Mux7/3
  [soc_sc_pcs] -> Mux9/1
  [vbus_pcs] -> 2/1
  2/1 -> MATLAB Function1/2(vbus_pcs), Mux5/3
  [vbus_vcs] -> 3/1
  [soc_pv2] -> Mux8/2
  [P_pv] -> Mux6/1
  [vbus_pv2] -> 4/1
  [soc_b_vcs] -> Mux8/4
  [P_pv2] -> Mux6/2
  Constant2/1 -> Mux6/4, Mux6/3
  [Soc_sc_vcs] -> Mux9/2
  [P_L1] -> Mux7/1
  Mux5/1 -> MATLAB Function1/1(V_bus)
  Mux6/1 -> MATLAB Function1/4(PV_power)
  Mux7/1 -> MATLAB Function1/5(Load_power)
  Mux8/1 -> MATLAB Function1/6(SoC_batt)
  Mux9/1 -> MATLAB Function1/7(SoC_sc)

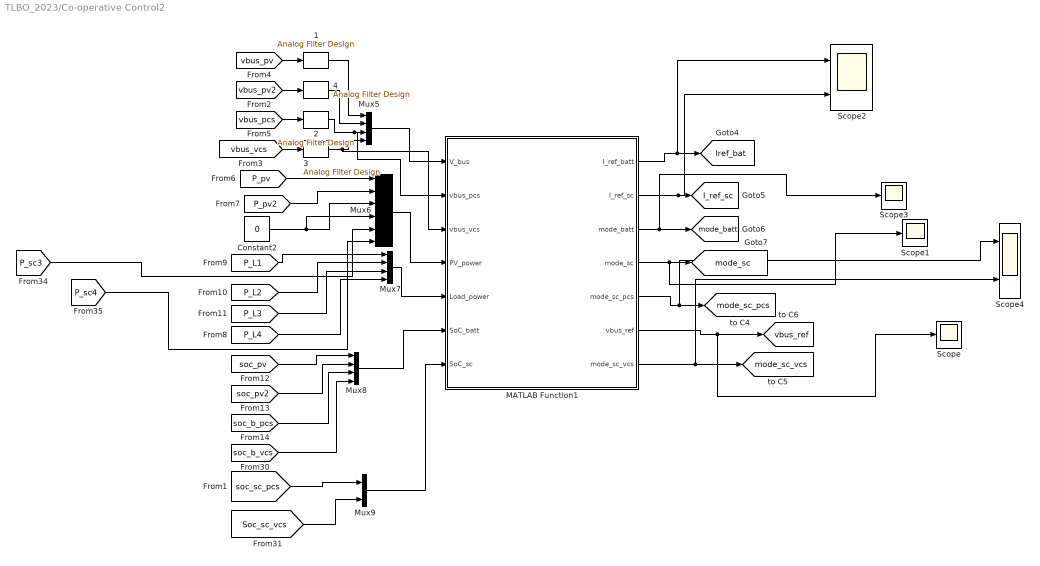
== system TLBO_2023/Co-operative Control2 ==
  {1..4} (4 alike) : dspfdesign/Analog Filter Design  method=Butterworth  filttype=Lowpass  N=8  Wlo=pi*50  Whi=80  Rp=2  Rs=40
  Constant2 : Constant  Value=0
  MATLAB Function1 : MATLAB Function  TreatAsAtomicUnit=on
  Mux5 : Mux
  Mux6 : Mux  Inputs=6
  Mux7 : Mux
  Mux8 : Mux
  Mux9 : Mux  Inputs=2
  Scope : Scope
  Scope1 : Scope
  Scope2 : Scope  NumInputPorts=2
  Scope3 : Scope
  Scope4 : Scope  NumInputPorts=2
  tag scope: I_ref_sc=global, Iref_bat=global, mode_batt=global, mode_sc=global, mode_sc_pcs=global, mode_sc_vcs=global, vbus_ref=global
  wires:
  Mux9/1 -> MATLAB Function1/7(SoC_sc)
  Mux8/1 -> MATLAB Function1/6(SoC_batt)
  Mux7/1 -> MATLAB Function1/5(Load_power)
  Mux6/1 -> MATLAB Function1/4(PV_power)
  Mux5/1 -> MATLAB Function1/1(V_bus)
  [P_L1] -> Mux7/1
  [Soc_sc_vcs] -> Mux9/2
  Constant2/1 -> Mux6/3, Mux6/4
  [P_pv2] -> Mux6/2
  [soc_b_vcs] -> Mux8/4
  [vbus_pv2] -> 4/1
  [P_pv] -> Mux6/1
  [soc_pv2] -> Mux8/2
  [vbus_vcs] -> 3/1
  2/1 -> Mux5/3, MATLAB Function1/2(vbus_pcs)
  [vbus_pcs] -> 2/1
  [soc_sc_pcs] -> Mux9/1
  [P_L3] -> Mux7/3
  3/1 -> Mux5/4, MATLAB Function1/3(vbus_vcs)
  [vbus_pv] -> 1/1
  [P_L2] -> Mux7/2
  [soc_b_pcs] -> Mux8/3
  1/1 -> Mux5/1
  [soc_pv] -> Mux8/1
  [P_L4] -> Mux7/4
  4/1 -> Mux5/2
  MATLAB Function1/1(I_ref_batt) -> [Iref_bat], Scope2/1
  [P_sc4] -> Mux6/6
  [P_sc3] -> Mux6/5
  MATLAB Function1/2(I_ref_sc) -> [I_ref_sc], Scope2/2
  MATLAB Function1/3(mode_batt) -> [mode_batt], Scope3/1
  MATLAB Function1/4(mode_sc) -> [mode_sc], Scope1/1
  MATLAB Function1/5(mode_sc_pcs) -> Scope4/1, [mode_sc_pcs]
  MATLAB Function1/7(mode_sc_vcs) -> Scope4/2, [mode_sc_vcs]
  MATLAB Function1/6(vbus_ref) -> [vbus_ref], Scope/1

== system TLBO_2023/Controller 2 ==
  Abs1 : Abs  SaturateOnIntegerOverflow=off
  Boost Battery1 : Switch  Criteria=u2 > Threshold  Threshold=0.5  SaturateOnIntegerOverflow=off  InputSameDT=off
  Buck Battery1 : Switch  Criteria=u2 > Threshold  Threshold=0.5  SaturateOnIntegerOverflow=off  InputSameDT=off
  Constant : Constant  Value=48
  Constant1 : Constant
  Constant2 : Constant  Value=2
  Constant3 : Constant  Value=0
  Constant4 : Constant  Value=0
  Local Controller : MATLAB Function  TreatAsAtomicUnit=on
  Logical Operator1 : Logic  Operator=NOT  AllPortsSameDT=off  OutDataTypeStr=boolean
  Null Gate1 : Constant  Value=0
  PID Controller3 : slpidlib/PID Controller  Controller=PI  Form=Parallel  TimeDomain=Discrete-time  UseExternalTs=off  SampleTime=-1  IntegratorMethod=Forward Euler  FilterMethod=Forward Euler  ControllerParametersSource=internal  P=0  I=4  UseKiTs=off  D=0  N=100  UseFilter=on  TunerSelectOption=Transfer Function Based (PID Tuner App)  InitialConditionSource=internal  InitialConditionForIntegrator=0  InitialConditionForFilter=0  DifferentiatorICPrevScaledInput=0  ExternalReset=none  TrackingMode=off  Kt=1  LimitOutput=off  SatLimitsSource=internal  UpperSaturationLimit=inf  LowerSaturationLimit=-inf  LinearizeAsGain=on  AntiWindupMode=none  Kb=1  LimitIntegrator=off  UpperIntegratorSaturationLimit=inf  LowerIntegratorSaturationLimit=-inf  POutMin=[]  POutMax=[]  IOutMin=[]  IOutMax=[]  DOutMin=[]  DOutMax=[]  NOutMin=[]  NOutMax=[]  SumOutMin=[]  SumOutMax=[]  SaturationOutMin=[]  SaturationOutMax=[]  PParamMin=[]  PParamMax=[]  IParamMin=[]  IParamMax=[]  DParamMin=[]  DParamMax=[]  NParamMin=[]  NParamMax=[]  KbParamMin=[]  KbParamMax=[]  KtParamMin=[]  KtParamMax=[]  KbOutMin=[]  KbOutMax=[]  KtOutMin=[]  KtOutMax=[]  IntegratorOutMin=[]  IntegratorOutMax=[]  FilterOutMin=[]  FilterOutMax=[]  SumI1OutMin=[]  SumI1OutMax=[]  SumI2OutMin=[]  SumI2OutMax=[]  SumI3OutMin=[]  SumI3OutMax=[]  SumI4OutMin=[]  SumI4OutMax=[]  SumDOutMin=[]  SumDOutMax=[]  DifferentiatorOutMin=[]  DifferentiatorOutMax=[]  FilterDiffOutCoefMin=[]  FilterDiffOutCoefMax=[]  ReciprocalOutMin=[]  ReciprocalOutMax=[]  SumDenOutMin=[]  SumDenOutMax=[]  SumNumOutMin=[]  SumNumOutMax=[]  DivideOutMin=[]  DivideOutMax=[]  UdiffTsProdOutMin=[]  UdiffTsProdOutMax=[]  NTsProdOutMin=[]  NTsProdOutMax=[]  UintegralTsProdOutMin=[]  UintegralTsProdOutMax=[]  UngainTsProdOutMin=[]  UngainTsProdOutMax=[]  ClampingZeroOutDataTypeStr=Inherit: Inherit via back propagation  ClampingZeroOutMin=[]  ClampingZeroOutMax=[]  FilterDenConstantOutDataTypeStr=Inherit: Inherit via back propagation  FilterDenConstantOutMin=[]  FilterDenConstantOutMax=[]  PCopyOutDataTypeStr=Inherit: Inherit via back propagation  PCopyOutMin=[]  PCopyOutMax=[]  NCopyOutDataTypeStr=Inherit: Inherit via back propagation  NCopyOutMin=[]  NCopyOutMax=[]  IntegratorContinuousStateAttributes=''  IntegratorStateMustResolveToSignalObject=off  IntegratorRTWStateStorageClass=Auto  FilterContinuousStateAttributes=''  FilterStateMustResolveToSignalObject=off  FilterRTWStateStorageClass=Auto  ParallelPVariant=InternalParameters  IdealPVariant=Disabled  IVariant=InternalParameters  DVariant=Disabled  IntegratorVariant=Discrete  SatVariant=Disabled  AWVariant=Passthrough  PCopyVariant=Disabled  TRVariant=Disabled  FdbkBlocksVariant=Forward  IdealPFdbkVariant=Disabled  SatFdbkVariant=Disabled  DerivativeFilterVariant=Disabled  NVariant=Disabled  NCopyVariant=Disabled_SignalSpec  FilterICVariant=Disabled  IntegratorICVariant=InternalICs  ExternalResetVariant=Disabled  TRSumVariant=Passthrough  SumFdbkVariant=Disabled  SumVariant=Sum_PI  TsampFilterVariant=InternalTs  TsampNgainVariant=Passthrough  TsampIntegralVariant=Disabled_SignalSpec  ExternalSaturationOutDataTypeStr=Inherit: Same as second input
  PID Controller5 : slpidlib/PID Controller  Controller=PI  Form=Parallel  TimeDomain=Discrete-time  UseExternalTs=off  SampleTime=-1  IntegratorMethod=Forward Euler  FilterMethod=Forward Euler  ControllerParametersSource=internal  P=10  I=4  UseKiTs=off  D=10  N=100  UseFilter=on  TunerSelectOption=Transfer Function Based (PID Tuner App)  InitialConditionSource=internal  InitialConditionForIntegrator=0  InitialConditionForFilter=0  DifferentiatorICPrevScaledInput=0  ExternalReset=none  TrackingMode=off  Kt=1  LimitOutput=off  SatLimitsSource=internal  UpperSaturationLimit=inf  LowerSaturationLimit=-inf  LinearizeAsGain=on  AntiWindupMode=none  Kb=1  LimitIntegrator=off  UpperIntegratorSaturationLimit=inf  LowerIntegratorSaturationLimit=-inf  POutMin=[]  POutMax=[]  IOutMin=[]  IOutMax=[]  DOutMin=[]  DOutMax=[]  NOutMin=[]  NOutMax=[]  SumOutMin=[]  SumOutMax=[]  SaturationOutMin=[]  SaturationOutMax=[]  PParamMin=[]  PParamMax=[]  IParamMin=[]  IParamMax=[]  DParamMin=[]  DParamMax=[]  NParamMin=[]  NParamMax=[]  KbParamMin=[]  KbParamMax=[]  KtParamMin=[]  KtParamMax=[]  KbOutMin=[]  KbOutMax=[]  KtOutMin=[]  KtOutMax=[]  IntegratorOutMin=[]  IntegratorOutMax=[]  FilterOutMin=[]  FilterOutMax=[]  SumI1OutMin=[]  SumI1OutMax=[]  SumI2OutMin=[]  SumI2OutMax=[]  SumI3OutMin=[]  SumI3OutMax=[]  SumI4OutMin=[]  SumI4OutMax=[]  SumDOutMin=[]  SumDOutMax=[]  DifferentiatorOutMin=[]  DifferentiatorOutMax=[]  FilterDiffOutCoefMin=[]  FilterDiffOutCoefMax=[]  ReciprocalOutMin=[]  ReciprocalOutMax=[]  SumDenOutMin=[]  SumDenOutMax=[]  SumNumOutMin=[]  SumNumOutMax=[]  DivideOutMin=[]  DivideOutMax=[]  UdiffTsProdOutMin=[]  UdiffTsProdOutMax=[]  NTsProdOutMin=[]  NTsProdOutMax=[]  UintegralTsProdOutMin=[]  UintegralTsProdOutMax=[]  UngainTsProdOutMin=[]  UngainTsProdOutMax=[]  ClampingZeroOutDataTypeStr=Inherit: Inherit via back propagation  ClampingZeroOutMin=[]  ClampingZeroOutMax=[]  FilterDenConstantOutDataTypeStr=Inherit: Inherit via back propagation  FilterDenConstantOutMin=[]  FilterDenConstantOutMax=[]  PCopyOutDataTypeStr=Inherit: Inherit via back propagation  PCopyOutMin=[]  PCopyOutMax=[]  NCopyOutDataTypeStr=Inherit: Inherit via back propagation  NCopyOutMin=[]  NCopyOutMax=[]  IntegratorContinuousStateAttributes=''  IntegratorStateMustResolveToSignalObject=off  IntegratorRTWStateStorageClass=Auto  FilterContinuousStateAttributes=''  FilterStateMustResolveToSignalObject=off  FilterRTWStateStorageClass=Auto  ParallelPVariant=InternalParameters  IdealPVariant=Disabled  IVariant=InternalParameters  DVariant=Disabled  IntegratorVariant=Discrete  SatVariant=Disabled  AWVariant=Passthrough  PCopyVariant=Disabled  TRVariant=Disabled  FdbkBlocksVariant=Forward  IdealPFdbkVariant=Disabled  SatFdbkVariant=Disabled  DerivativeFilterVariant=Disabled  NVariant=Disabled  NCopyVariant=Disabled_SignalSpec  FilterICVariant=Disabled  IntegratorICVariant=InternalICs  ExternalResetVariant=Disabled  TRSumVariant=Passthrough  SumFdbkVariant=Disabled  SumVariant=Sum_PI  TsampFilterVariant=InternalTs  TsampNgainVariant=Passthrough  TsampIntegralVariant=Disabled_SignalSpec  ExternalSaturationOutDataTypeStr=Inherit: Same as second input
  PWM Generator (DC-DC)2 : spsPWMGeneratorDCDCLib/PWM Generator (DC-DC)  Fsw=10e3  Ts=0
  P_b3 : Display
      settings: Format=binary (Stored Integer)  Decimation=1000
  Reshape : Reshape
  Saturation : Saturate
  Saturation1 : Saturate  UpperLimit=0.8  LowerLimit=0  ZeroCross=off
  Scope1 : Scope
  Scope2 : Scope
  Scope5 : Scope
  Subtract1 : Sum
  Subtract2 : Sum  Inputs=+-
  Subtract4 : Sum  Inputs=+-
  Variable Selector : dspindex/Variable Selector  NumInputs=1  rowsOrCols=Rows  IdxMode=Variable  Elements=[1 3]  ZerOneIdxMode=One-based  errmode=Clip Index  FillMode=on  FillValues=0
  Variable Selector1 : dspindex/Variable Selector  NumInputs=1  rowsOrCols=Columns  IdxMode=Variable  Elements=[1 3]  ZerOneIdxMode=One-based  errmode=Clip Index  FillMode=on  FillValues=0
  tag scope: boost_b_pv2=global, buck_b_pv2=global
  wires:
  Buck Battery1/1 -> [buck_b_pv2]
  Boost Battery1/1 -> [boost_b_pv2]
  Null Gate1/1 -> Boost Battery1/3, Buck Battery1/3
  [vbus_pv2] -> Local Controller/1(vbus_pv2)
  Subtract2/1 -> Abs1/1
  Logical Operator1/1 -> Buck Battery1/2
  Local Controller/1(b_control) -> Scope2/1, P_b3/1, Logical Operator1/1, Boost Battery1/2
  [vbus_pv2] -> Subtract2/1
  Abs1/1 -> PID Controller3/1
  PWM Generator (DC-DC)2/1 -> Buck Battery1/1, Boost Battery1/1
  PID Controller5/1 -> Saturation1/1
  Saturation1/1 -> Scope1/1, PWM Generator (DC-DC)2/1
  Subtract4/1 -> Scope5/1, PID Controller5/1
  [ib_pv2] -> Subtract4/2
  [vbus_ref] -> Local Controller/2(vbus_ref)
  Constant/1 -> Subtract2/2
  Reshape/1 -> Saturation/1
  Constant1/1 -> Variable Selector/2
  Variable Selector1/1 -> Reshape/1
  [Iref_bat] -> Variable Selector/1
  Variable Selector/1 -> Variable Selector1/1
  Constant2/1 -> Variable Selector1/2
  PID Controller3/1 -> Subtract1/1
  Subtract1/1 -> Subtract4/1
  Saturation/1 -> Subtract1/2
  Constant4/1 -> Local Controller/3(mode_pv2)

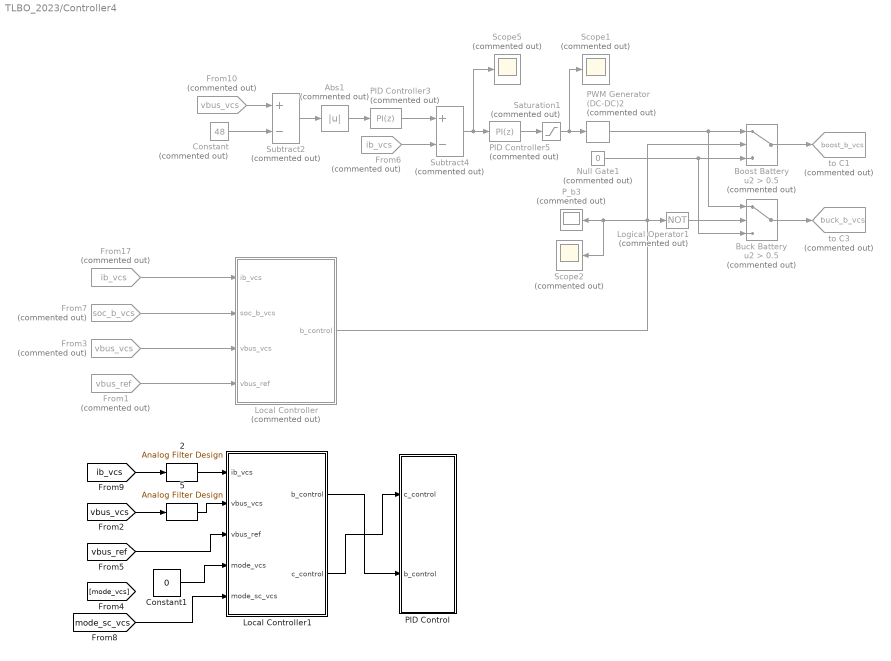
== system TLBO_2023/Controller4 ==
  2 : dspfdesign/Analog Filter Design  method=Butterworth  filttype=Lowpass  N=8  Wlo=pi*50  Whi=80  Rp=2  Rs=40
  5 : dspfdesign/Analog Filter Design  method=Butterworth  filttype=Lowpass  N=8  Wlo=pi*50  Whi=80  Rp=2  Rs=40
  Abs1 : Abs  Commented=on  SaturateOnIntegerOverflow=off
  Boost Battery : Switch  Commented=on  Criteria=u2 > Threshold  Threshold=0.5  SaturateOnIntegerOverflow=off  InputSameDT=off
  Buck Battery : Switch  Commented=on  Criteria=u2 > Threshold  Threshold=0.5  SaturateOnIntegerOverflow=off  InputSameDT=off
  Constant : Constant  Commented=on  Value=48
  Constant1 : Constant  Value=0
  From1 : From  Commented=on  GotoTag=vbus_ref  TagVisibility=global
  From10 : From  Commented=on  GotoTag=vbus_vcs  TagVisibility=global
  From17 : From  Commented=on  GotoTag=ib_vcs  TagVisibility=global
  From3 : From  Commented=on  GotoTag=vbus_vcs  TagVisibility=global
  From6 : From  Commented=on  GotoTag=ib_vcs  TagVisibility=global
  From7 : From  Commented=on  GotoTag=soc_b_vcs  TagVisibility=global
  Local Controller : MATLAB Function  Commented=on  TreatAsAtomicUnit=on
  Local Controller1 : MATLAB Function  TreatAsAtomicUnit=on
  Logical Operator1 : Logic  Commented=on  Operator=NOT  AllPortsSameDT=off  OutDataTypeStr=boolean
  Null Gate1 : Constant  Commented=on  Value=0
  PID Control : Subsystem
  PID Controller3 : slpidlib/PID Controller  Commented=on  Controller=PI  Form=Parallel  TimeDomain=Discrete-time  UseExternalTs=off  SampleTime=-1  IntegratorMethod=Forward Euler  FilterMethod=Forward Euler  ControllerParametersSource=internal  P=0  I=4  UseKiTs=off  D=0  N=100  UseFilter=on  TunerSelectOption=Transfer Function Based (PID Tuner App)  InitialConditionSource=internal  InitialConditionForIntegrator=0  InitialConditionForFilter=0  DifferentiatorICPrevScaledInput=0  ExternalReset=none  TrackingMode=off  Kt=1  LimitOutput=off  SatLimitsSource=internal  UpperSaturationLimit=inf  LowerSaturationLimit=-inf  LinearizeAsGain=on  AntiWindupMode=none  Kb=1  LimitIntegrator=off  UpperIntegratorSaturationLimit=inf  LowerIntegratorSaturationLimit=-inf  POutMin=[]  POutMax=[]  IOutMin=[]  IOutMax=[]  DOutMin=[]  DOutMax=[]  NOutMin=[]  NOutMax=[]  SumOutMin=[]  SumOutMax=[]  SaturationOutMin=[]  SaturationOutMax=[]  PParamMin=[]  PParamMax=[]  IParamMin=[]  IParamMax=[]  DParamMin=[]  DParamMax=[]  NParamMin=[]  NParamMax=[]  KbParamMin=[]  KbParamMax=[]  KtParamMin=[]  KtParamMax=[]  KbOutMin=[]  KbOutMax=[]  KtOutMin=[]  KtOutMax=[]  IntegratorOutMin=[]  IntegratorOutMax=[]  FilterOutMin=[]  FilterOutMax=[]  SumI1OutMin=[]  SumI1OutMax=[]  SumI2OutMin=[]  SumI2OutMax=[]  SumI3OutMin=[]  SumI3OutMax=[]  SumI4OutMin=[]  SumI4OutMax=[]  SumDOutMin=[]  SumDOutMax=[]  DifferentiatorOutMin=[]  DifferentiatorOutMax=[]  FilterDiffOutCoefMin=[]  FilterDiffOutCoefMax=[]  ReciprocalOutMin=[]  ReciprocalOutMax=[]  SumDenOutMin=[]  SumDenOutMax=[]  SumNumOutMin=[]  SumNumOutMax=[]  DivideOutMin=[]  DivideOutMax=[]  UdiffTsProdOutMin=[]  UdiffTsProdOutMax=[]  NTsProdOutMin=[]  NTsProdOutMax=[]  UintegralTsProdOutMin=[]  UintegralTsProdOutMax=[]  UngainTsProdOutMin=[]  UngainTsProdOutMax=[]  ClampingZeroOutDataTypeStr=Inherit: Inherit via back propagation  ClampingZeroOutMin=[]  ClampingZeroOutMax=[]  FilterDenConstantOutDataTypeStr=Inherit: Inherit via back propagation  FilterDenConstantOutMin=[]  FilterDenConstantOutMax=[]  PCopyOutDataTypeStr=Inherit: Inherit via back propagation  PCopyOutMin=[]  PCopyOutMax=[]  NCopyOutDataTypeStr=Inherit: Inherit via back propagation  NCopyOutMin=[]  NCopyOutMax=[]  IntegratorContinuousStateAttributes=''  IntegratorStateMustResolveToSignalObject=off  IntegratorRTWStateStorageClass=Auto  FilterContinuousStateAttributes=''  FilterStateMustResolveToSignalObject=off  FilterRTWStateStorageClass=Auto  ParallelPVariant=InternalParameters  IdealPVariant=Disabled  IVariant=InternalParameters  DVariant=Disabled  IntegratorVariant=Discrete  SatVariant=Disabled  AWVariant=Passthrough  PCopyVariant=Disabled  TRVariant=Disabled  FdbkBlocksVariant=Forward  IdealPFdbkVariant=Disabled  SatFdbkVariant=Disabled  DerivativeFilterVariant=Disabled  NVariant=Disabled  NCopyVariant=Disabled_SignalSpec  FilterICVariant=Disabled  IntegratorICVariant=InternalICs  ExternalResetVariant=Disabled  TRSumVariant=Passthrough  SumFdbkVariant=Disabled  SumVariant=Sum_PI  TsampFilterVariant=InternalTs  TsampNgainVariant=Passthrough  TsampIntegralVariant=Disabled_SignalSpec  ExternalSaturationOutDataTypeStr=Inherit: Same as second input
  PID Controller5 : slpidlib/PID Controller  Commented=on  Controller=PI  Form=Parallel  TimeDomain=Discrete-time  UseExternalTs=off  SampleTime=-1  IntegratorMethod=Forward Euler  FilterMethod=Forward Euler  ControllerParametersSource=internal  P=1  I=4  UseKiTs=off  D=1  N=100  UseFilter=on  TunerSelectOption=Transfer Function Based (PID Tuner App)  InitialConditionSource=internal  InitialConditionForIntegrator=0  InitialConditionForFilter=0  DifferentiatorICPrevScaledInput=0  ExternalReset=none  TrackingMode=off  Kt=1  LimitOutput=off  SatLimitsSource=internal  UpperSaturationLimit=inf  LowerSaturationLimit=-inf  LinearizeAsGain=on  AntiWindupMode=none  Kb=1  LimitIntegrator=off  UpperIntegratorSaturationLimit=inf  LowerIntegratorSaturationLimit=-inf  POutMin=[]  POutMax=[]  IOutMin=[]  IOutMax=[]  DOutMin=[]  DOutMax=[]  NOutMin=[]  NOutMax=[]  SumOutMin=[]  SumOutMax=[]  SaturationOutMin=[]  SaturationOutMax=[]  PParamMin=[]  PParamMax=[]  IParamMin=[]  IParamMax=[]  DParamMin=[]  DParamMax=[]  NParamMin=[]  NParamMax=[]  KbParamMin=[]  KbParamMax=[]  KtParamMin=[]  KtParamMax=[]  KbOutMin=[]  KbOutMax=[]  KtOutMin=[]  KtOutMax=[]  IntegratorOutMin=[]  IntegratorOutMax=[]  FilterOutMin=[]  FilterOutMax=[]  SumI1OutMin=[]  SumI1OutMax=[]  SumI2OutMin=[]  SumI2OutMax=[]  SumI3OutMin=[]  SumI3OutMax=[]  SumI4OutMin=[]  SumI4OutMax=[]  SumDOutMin=[]  SumDOutMax=[]  DifferentiatorOutMin=[]  DifferentiatorOutMax=[]  FilterDiffOutCoefMin=[]  FilterDiffOutCoefMax=[]  ReciprocalOutMin=[]  ReciprocalOutMax=[]  SumDenOutMin=[]  SumDenOutMax=[]  SumNumOutMin=[]  SumNumOutMax=[]  DivideOutMin=[]  DivideOutMax=[]  UdiffTsProdOutMin=[]  UdiffTsProdOutMax=[]  NTsProdOutMin=[]  NTsProdOutMax=[]  UintegralTsProdOutMin=[]  UintegralTsProdOutMax=[]  UngainTsProdOutMin=[]  UngainTsProdOutMax=[]  ClampingZeroOutDataTypeStr=Inherit: Inherit via back propagation  ClampingZeroOutMin=[]  ClampingZeroOutMax=[]  FilterDenConstantOutDataTypeStr=Inherit: Inherit via back propagation  FilterDenConstantOutMin=[]  FilterDenConstantOutMax=[]  PCopyOutDataTypeStr=Inherit: Inherit via back propagation  PCopyOutMin=[]  PCopyOutMax=[]  NCopyOutDataTypeStr=Inherit: Inherit via back propagation  NCopyOutMin=[]  NCopyOutMax=[]  IntegratorContinuousStateAttributes=''  IntegratorStateMustResolveToSignalObject=off  IntegratorRTWStateStorageClass=Auto  FilterContinuousStateAttributes=''  FilterStateMustResolveToSignalObject=off  FilterRTWStateStorageClass=Auto  ParallelPVariant=InternalParameters  IdealPVariant=Disabled  IVariant=InternalParameters  DVariant=Disabled  IntegratorVariant=Discrete  SatVariant=Disabled  AWVariant=Passthrough  PCopyVariant=Disabled  TRVariant=Disabled  FdbkBlocksVariant=Forward  IdealPFdbkVariant=Disabled  SatFdbkVariant=Disabled  DerivativeFilterVariant=Disabled  NVariant=Disabled  NCopyVariant=Disabled_SignalSpec  FilterICVariant=Disabled  IntegratorICVariant=InternalICs  ExternalResetVariant=Disabled  TRSumVariant=Passthrough  SumFdbkVariant=Disabled  SumVariant=Sum_PI  TsampFilterVariant=InternalTs  TsampNgainVariant=Passthrough  TsampIntegralVariant=Disabled_SignalSpec  ExternalSaturationOutDataTypeStr=Inherit: Same as second input
  PWM Generator (DC-DC)2 : spsPWMGeneratorDCDCLib/PWM Generator (DC-DC)  Commented=on  Fsw=10e3  Ts=0
  P_b3 : Display  Commented=on
      settings: Format=binary (Stored Integer)  Decimation=1000
  Saturation1 : Saturate  Commented=on  UpperLimit=0.8  LowerLimit=0  ZeroCross=off
  Scope1 : Scope  Commented=on
  Scope2 : Scope  Commented=on
  Scope5 : Scope  Commented=on
  Subtract2 : Sum  Commented=on  Inputs=+-
  Subtract4 : Sum  Commented=on  Inputs=+-
  to C1 : Goto  Commented=on  GotoTag=boost_b_vcs  TagVisibility=global
  to C3 : Goto  Commented=on  GotoTag=buck_b_vcs  TagVisibility=global
  wires:
  Buck Battery/1 -> to C3/1
  Boost Battery/1 -> to C1/1
  Null Gate1/1 -> Boost Battery/3, Buck Battery/3
  From17/1 -> Local Controller/1(ib_vcs)
  From3/1 -> Local Controller/3(vbus_vcs)
  From7/1 -> Local Controller/2(soc_b_vcs)
  Subtract2/1 -> Abs1/1
  Logical Operator1/1 -> Buck Battery/2
  Local Controller/1(b_control) -> Scope2/1, P_b3/1, Logical Operator1/1, Boost Battery/2
  From10/1 -> Subtract2/1
  Abs1/1 -> PID Controller3/1
  PWM Generator (DC-DC)2/1 -> Buck Battery/1, Boost Battery/1
  PID Controller5/1 -> Saturation1/1
  Saturation1/1 -> Scope1/1, PWM Generator (DC-DC)2/1
  Subtract4/1 -> Scope5/1, PID Controller5/1
  PID Controller3/1 -> Subtract4/1
  From6/1 -> Subtract4/2
  From1/1 -> Local Controller/4(vbus_ref)
  Constant/1 -> Subtract2/2
  [vbus_vcs] -> 5/1
  [ib_vcs] -> 2/1
  [vbus_ref] -> Local Controller1/3(vbus_ref)
  5/1 -> Local Controller1/2(vbus_vcs)
  2/1 -> Local Controller1/1(ib_vcs)
  Local Controller1/1(b_control) -> PID Control/2(b_control)
  Local Controller1/2(c_control) -> PID Control/1(c_control)
  [mode_sc_vcs] -> Local Controller1/5(mode_sc_vcs)
  Constant1/1 -> Local Controller1/4(mode_vcs)
